simulink model "MASc_AndriyPredmyrskyy_SAC"  (R2020a)
settings: Solver=FixedStepAuto  StartTime=0.0  StopTime=tsim  FixedStep=baseRate  RelTol=1e-3  EnableMultiTasking=on
values from neighbouring files (symbols this model uses):
  Amp1off = 0.2    [Run_Initializer.m]
  Amp2off = 0.1    [Run_Initializer.m]
  baseRate = 0.05    [Run_Initializer.m]
  BLACKMass = 12.3341    [LoadResults.m]    (also in Run_Initializer.m = model_param(3))
  Cmout = [eye(3,3),zeros(3,3)]    [Run_Initializer.m]    (also in SimpleSAC.m = [alpha*eye(3,3),eye(3,3)])
  D = 0    [OptimizationPlots.m]    (also in OptimizeSAC_DE.m; OptimizeSAC_DE_CHANGE.m; OptimizeSAC_PSO.m; SADE_OptimizationForSAC.m)
  drop_states_BLACK = [2.3,1.5,0.176047682762146]    [Run_Initializer.m]
  drop_states_BLUE = [ xLength/2+0.9; yLength/2+0.5; 0]    [Run_Initializer.m]
  drop_states_RED = [2.60644311523438,1.21791186523438,3.08142089843750]    [Run_Initializer.m]
  F_thrusters_BLACK = 0.25.*ones(8,1)    [Run_Initializer.m]
  F_thrusters_BLUE = 0.25.*ones(8,1)    [Run_Initializer.m]
  F_thrusters_RED = 0.25.*ones(8,1)    [Run_Initializer.m]
  GeI = X(2,Best_i).*eye(3)    [OptimizeSAC_DE.m]    (also in OptimizeSAC_DE_CHANGE.m; OptimizeSAC_PSO.m = pos(besti,5).*eye(3); RunAllOptimizations.m = Init.GeI; SADE_OptimizationForSAC.m)
  GeP = X(1,Best_i).*eye(3)    [OptimizeSAC_DE.m]    (also in OptimizeSAC_DE_CHANGE.m; OptimizeSAC_PSO.m = pos(besti,1).*eye(3); RunAllOptimizations.m = Init.GeP; SADE_OptimizationForSAC.m)
  GuI = X(4,Best_i).*eye(3)    [OptimizeSAC_DE.m]    (also in OptimizeSAC_DE_CHANGE.m; OptimizeSAC_PSO.m = pos(besti,8).*eye(3); RunAllOptimizations.m = Init.GuI; SADE_OptimizationForSAC.m)
  GuP = X(3,Best_i).*eye(3)    [OptimizeSAC_DE.m]    (also in OptimizeSAC_DE_CHANGE.m; OptimizeSAC_PSO.m = pos(besti,4).*eye(3); RunAllOptimizations.m = Init.GuP; SADE_OptimizationForSAC.m)
  GxI = blkdiag(X(7,Best_i).*eye(3),X(8,Best_i).*eye(3))    [OptimizeSAC_DE.m]    (also in OptimizeSAC_DE_CHANGE.m = X(6,Best_i).*eye(6); OptimizeSAC_PSO.m = blkdiag(pos(besti,6).*eye(3),pos(besti,7).*eye(3)); RunAllOptimizations.m = Init.GxI; SADE_OptimizationForSAC.m)
  GxP = blkdiag(X(5,Best_i).*eye(3),X(6,Best_i).*eye(3))    [OptimizeSAC_DE.m]    (also in OptimizeSAC_DE_CHANGE.m = X(5,Best_i).*eye(6); OptimizeSAC_PSO.m = blkdiag(pos(besti,2).*eye(3),pos(besti,3).*eye(3)); RunAllOptimizations.m = Init.GxP; SADE_OptimizationForSAC.m)
  GzI = 1e0.*eye(12)    [Run_Initializer.m]
  GzP = 0e-2.*eye(12)    [Run_Initializer.m]
  home_states_BLACK = LastPosition    [Run_Initializer.m]
  home_states_BLUE = [ xLength/2-0.9; yLength/2+0.5; 0]    [Run_Initializer.m]
  home_states_RED = [ xLength/2+0.7; yLength/2; 0]    [Run_Initializer.m]
  init_states_BLACK = FirstPosition    [Run_Initializer.m]
  init_states_BLUE = [ xLength/2+0.9; yLength/2+0.5; 0]    [Run_Initializer.m]
  init_states_RED = [ xLength/2+0.7; yLength/2; 0]    [Run_Initializer.m]
  K = 3    [Run_Initializer.m]    (also in cycloid.m)
  K_Force = 1    [Run_Initializer.m]
  Kd_Force = 3    [Run_Initializer.m]
  Kd_tb = 0.4    [Run_Initializer.m]
  Kd_tblue = 0.4    [Run_Initializer.m]
  Kd_tr = 0.4    [Run_Initializer.m]
  Kd_xb = 5    [Run_Initializer.m]
  Kd_xblue = 5    [Run_Initializer.m]
  Kd_xr = 5    [Run_Initializer.m]
  Kd_yb = 5    [Run_Initializer.m]
  Kd_yblue = 5    [Run_Initializer.m]
  Kd_yr = 5    [Run_Initializer.m]
  KeI0 = 0.*[   0.1063   -0.0058         0 ... (first row only)    [Run_Initializer.m]    (also in SimpleSAC.m = zeros(3))
  Kp_tb = 0.1    [Run_Initializer.m]
  Kp_tblue = 0.1    [Run_Initializer.m]
  Kp_tr = 0.1    [Run_Initializer.m]
  Kp_xb = 2    [Run_Initializer.m]
  Kp_xblue = 2    [Run_Initializer.m]
  Kp_xr = 2    [Run_Initializer.m]
  Kp_yb = 2    [Run_Initializer.m]
  Kp_yblue = 2    [Run_Initializer.m]
  Kp_yr = 2    [Run_Initializer.m]
  KuI0 = 0.*0.2193*[1,0,0;0,1,0;0,0,0]    [Run_Initializer.m]    (also in SimpleSAC.m = zeros(3))
  KxI0 = 0.*[-0.2193*eye(3),-3.2891*eye(3)]    [Run_Initializer.m]    (also in SimpleSAC.m = zeros(3,6))
  KzI0 = zeros(3,12)    [Run_Initializer.m]
  noise_variance_BLACK = 0    [Run_Initializer.m]
  noise_variance_BLUE = 0    [Run_Initializer.m]
  noise_variance_RED = 0    [Run_Initializer.m]
  omega = 0.03    [LoadResults.m]    (also in OptimizeSAC_PSO.m = 0.2; Run_Initializer.m = 0.06; SPSO_OptimizationForSAC.m = 0.2; SimpleSAC.m = sqrt(Force./(Mass*Radius)))
  omega1off = 0.03    [Run_Initializer.m]
  omega2off = 0.06    [Run_Initializer.m]
  Phase0_End = Phase0_Duration    (= 10)    [Run_Initializer.m]
  Phase1_End = Phase0_Duration + Phase1_Duration    (= 15)    [Run_Initializer.m]
  phase1off = 2*pi + 3-2+1.0654    (= 8.34858530718)    [Run_Initializer.m]
  Phase2_End = Phase0_Duration + Phase1_Duration +                                   Phase2_Duration    (= 35)    [Run_Initializer.m]
  phase2off = mod(pi^66,2*pi)    [Run_Initializer.m]
  Phase3_End = Phase0_Duration + Phase1_Duration +                                   Phase2_Duration + Phase3_Duration    (= 246)    [Run_Initializer.m]
  Phase3_SubPhase1_End = Phase2_End + Phase3_SubPhase1_Duration    (= 40)    [Run_Initializer.m]
  Phase3_SubPhase2_End = Phase2_End + Phase3_SubPhase1_Duration +                                   Phase3_SubPhase2_Duration    (= 45)    [Run_Initializer.m]
  Phase3_SubPhase3_End = Phase2_End + Phase3_SubPhase1_Duration +                                   Phase3_SubPhase2_Duration +                                  Phase3_SubPhase3_Duration    (= 46)    [Run_Initializer.m]
  Phase3_SubPhase4_End = Phase2_End + Phase3_SubPhase1_Duration +                                   Phase3_SubPhase2_Duration +                                  Phase3_SubPhase3_Duration +                                  Phase3_SubPhase4_Duration    [Run_Initializer.m]
  Phase4_End = Phase0_Duration + Phase1_Duration +                                   Phase2_Duration + Phase3_Duration +                                   Phase4_Duration    (= 266)    [Run_Initializer.m]
  Phase5_End = Phase0_Duration + Phase1_Duration +                                   Phase2_Duration + Phase3_Duration +                                   Phase4_Duration + Phase5_Duration    (= 271)    [Run_Initializer.m]
  platformSelection = 1    [OptimizationPlots.m]    (also in OptimizeSAC_DE.m; OptimizeSAC_DE_CHANGE.m; OptimizeSAC_PSO.m; SADE_OptimizationForSAC.m)
  serverRate = 0.1    [Run_Initializer.m]    (also in SimpleSAC.m)
  sigma_eI = X(9,Best_i)    [OptimizeSAC_DE.m]    (also in OptimizeSAC_DE_CHANGE.m = X(7,Best_i); OptimizeSAC_PSO.m = pos(besti,9); RunAllOptimizations.m = Init.sigma_eI; SADE_OptimizationForSAC.m)
  sigma_uI = X(10,Best_i)    [OptimizeSAC_DE.m]    (also in OptimizeSAC_DE_CHANGE.m = X(8,Best_i); OptimizeSAC_PSO.m = pos(besti,11); RunAllOptimizations.m = Init.sigma_uI; SADE_OptimizationForSAC.m)
  sigma_xI = X(11,Best_i)    [OptimizeSAC_DE.m]    (also in OptimizeSAC_DE_CHANGE.m = X(9,Best_i); OptimizeSAC_PSO.m = pos(besti,10); RunAllOptimizations.m = Init.sigma_xI; SADE_OptimizationForSAC.m)
  sigma_zI = 0    [Run_Initializer.m]
  sysd1 = c2d(sys,baseRate,opt)    [Run_Initializer.m]    (also in SimpleSAC.m = c2d(sys,serverRate,opt))
  sysd2 = c2d(sysInverse,baseRate,opt)    [Run_Initializer.m]
  thruster_dist2CG_BLACK = [83.42;-52.58;55.94;-60.05;54.08;-53.92;77.06;-55.94]    [Run_Initializer.m]
  thruster_dist2CG_BLUE = [83.42;-52.58;55.94;-60.05;54.08;-53.92;77.06;-55.94]    [Run_Initializer.m]
  thruster_dist2CG_RED = [49.92;-78.08;70.46;-63.54;81.08;-50.42;57.44;-75.96]    [Run_Initializer.m]
  xm2_ini = -(sysd2.D(1,1).*xm_ini(1:3))./(sysd2.C(1,1))    [Run_Initializer.m]
  xm_ini = [FirstPosition(1), FirstPosition(2), 0, 0, 0, 0]'    [Run_Initializer.m]    (also in SimpleSAC.m = [0, 0, 0, 0, 0, 0]')
undefined symbols (not defined in the file or in its folder): DiscIntNeverNeededParam, G3, simMode, WhoAmI
libraries: dspstat3 x18, simulink x12, raspberrypiBasiclib x10, dspsigops x9, embdlinuxlib x8, mspfiltlib x3, dsparch4 x3, peGeneralControl x3, eeGeneralControl x3, dspswit3 x2, MainLibrary x2, sensehatlib x1
(part 11 of 11)

== matlab function MASc_AndriyPredmyrskyy_SAC/From Torque, Command RW/Change RED Behavior/Calculate Saturated RPM Signal/Calculate RW RPM Increment ==
  data: Tz_Sat input; dRPM_RW output
function dRPM_RW = Calc_RW_RPM(Tz_Sat)

dRPM_RW =  (Tz_Sat/0.007244720)*(60/2/pi)*0.1;

end

== matlab function MASc_AndriyPredmyrskyy_SAC/From Torque, Command RW/Change RED Behavior/Wheel RPM to PWM/Check if RW is Ready ==
  data: Status input; EnableSig output; WheelRPM_In input; WheelRPM_Out output
function [EnableSig, WheelRPM_Out] = Check_Wheel_Status(Status, WheelRPM_In)

if Status == 0
    EnableSig    = 1;
    WheelRPM_Out = WheelRPM_In;
else
    EnableSig    = 0;
    WheelRPM_Out = 0;
end

end

== matlab function MASc_AndriyPredmyrskyy_SAC/From Torque, Command RW/Change RED Behavior/Wheel RPM to PWM/Get RW Direction ==
  data: MotorRPM_Sat input; WheelDirection output
function WheelDirection = GetDirection(MotorRPM_Sat)

if MotorRPM_Sat > 0
    WheelDirection = 0;
else
    WheelDirection = 1;
end
        
end

== matlab function MASc_AndriyPredmyrskyy_SAC/From Torque, Command RW/Change RED Behavior/Wheel RPM to PWM/RPM to PWM Value ==
  data: MotorRPM_Sat input; MotorPWM output
function MotorPWM = RPM2PWM(MotorRPM_Sat)

PWMRange = 0.9-0.1;

MotorPWM = ((MotorRPM_Sat*PWMRange)/7000) + 0.1;

end

== matlab function MASc_AndriyPredmyrskyy_SAC/Phase #3: Experiment/Change RED Behavior/Sub-Phase #4/MATLAB Function ==
  data: t input; x output; xLength parameter
function x = fcn(t, xLength)

x = 0.7*cos((0.104719755/2)*t) + xLength/2;

end

== matlab function MASc_AndriyPredmyrskyy_SAC/From Force//Torque to PWM Signal/Change BLUE Behavior/Calculate Thruster ON//OFF/MATLAB Function ==
  data: H output; thruster_dist2CG_BLUE parameter; F_thrusters_BLUE parameter
function H = MakeH(thruster_dist2CG_BLUE,F_thrusters_BLUE)

Vec1 = [ -1
         -1
          0 
          0
          1
          1
          0
          0 ];
      
Vec2 = [  0
          0
          1
          1
          0
          0
         -1
         -1 ];
     
Vec3 = thruster_dist2CG_BLUE./1000;

Mat1 = [Vec1, Vec2, Vec3]';

Mat2 = diag((F_thrusters_BLUE./2));

H    = Mat1*Mat2;

end

== matlab function MASc_AndriyPredmyrskyy_SAC/Phase #3: Experiment/Change RED Behavior/Sub-Phase #4/MATLAB Function1 ==
  data: t input; y output; yLength parameter
function y = fcn(t, yLength)

y = 0.7*sin((0.104719755/2)*t) + yLength/2;

end

== matlab function MASc_AndriyPredmyrskyy_SAC/Phase #3: Experiment/Change BLACK Behavior/Sub-Phase #4/Hough Control/MATLAB Function4 ==
  data: Oy input; e_out output; e_in input
function e_out = fcn(Oy, e_in)

a = sign(Oy'*e_in);
e_out = -a*norm(e_in);

== matlab function MASc_AndriyPredmyrskyy_SAC/Gyroscope & Acceleration Algorithms/Change RED Behavior/Create Rotation Matrix ==
  data: Rz input; C_Ib output
function C_Ib = RotateFrame(Rz)

C_bI = [  cos(Rz) sin(Rz)
         -sin(Rz) cos(Rz) ];

C_Ib = inv(C_bI);

end

== matlab function MASc_AndriyPredmyrskyy_SAC/Gyroscope & Acceleration Algorithms/Change BLACK Behavior/Create Rotation Matrix ==
  data: Rz input; C_Ib output
function C_Ib = RotateFrame(Rz)

C_bI = [  cos(Rz) sin(Rz)
         -sin(Rz) cos(Rz) ];

C_Ib = inv(C_bI);

end

== matlab function MASc_AndriyPredmyrskyy_SAC/Gyroscope & Acceleration Algorithms/Change RED Behavior/ChangeOrientation ==
  data: u input; y output
function y = ChangeOrientation(u)

y = rotz(-90)*u';

== matlab function MASc_AndriyPredmyrskyy_SAC/Gyroscope & Acceleration Algorithms/Change BLACK Behavior/ChangeOrientation ==
  data: u input; y output
function y = ChangeOrientation(u)

y = rotz(-90)*u';

== matlab function MASc_AndriyPredmyrskyy_SAC/Gyroscope & Acceleration Algorithms/Change BLUE Behavior/ChangeOrientation ==
  data: u input; y output
function y = ChangeOrientation(u)

y = rotz(-90)*u';

== matlab function MASc_AndriyPredmyrskyy_SAC/Gyroscope & Acceleration Algorithms/Change BLUE Behavior/Create Rotation Matrix ==
  data: Rz input; C_Ib output
function C_Ib = RotateFrame(Rz)

C_bI = [  cos(Rz) sin(Rz)
         -sin(Rz) cos(Rz) ];

C_Ib = inv(C_bI);

end

== matlab function MASc_AndriyPredmyrskyy_SAC/From Force//Torque to PWM Signal/Change BLUE Behavior/Calculate Thruster ON//OFF/MATLAB Function1 ==
  data: H output; thruster_dist2CG_BLUE parameter; F_thrusters_BLUE parameter
function H = MakeH(thruster_dist2CG_BLUE,F_thrusters_BLUE)

Vec1 = [ -1
         -1
          0 
          0
          1
          1
          0
          0 ];
      
Vec2 = [  0
          0
          1
          1
          0
          0
         -1
         -1 ];
     
Vec3 = thruster_dist2CG_BLUE./1000;

Mat1 = [Vec1, Vec2, Vec3]';

Mat2 = diag((F_thrusters_BLUE./2));

H    = Mat1*Mat2;

end

== matlab function MASc_AndriyPredmyrskyy_SAC/From Force//Torque to PWM Signal/Change BLUE Behavior/Calculate Thruster ON//OFF/MATLAB Function2 ==
  data: ThrustPer_Final output; ThrustPer input
function ThrustPer_Final  = ThrusterSat(ThrustPer)

ValveTime       = 0.007;
TControl        = 0.1;
ThrustPer_Final = zeros(8,1);

if max(ThrustPer) > 1
    ThrustPer_Sat = ThrustPer/max(ThrustPer);
else
    ThrustPer_Sat = ThrustPer;
end

for i = 1:8
    if ThrustPer_Sat(i) > ValveTime/TControl 
        ThrustPer_Final(i) = ThrustPer_Sat(i);
    else
        ThrustPer_Final(i) = 0;
    end
end
   

end

== matlab function MASc_AndriyPredmyrskyy_SAC/From Force//Torque to PWM Signal/Change BLUE Behavior/Calculate Thruster ON//OFF/Rotate Forces to Inertial/Create Rotation Matrix ==
  data: Rz input; C_Ib output
function C_Ib = RotateFrame(Rz)

C_bI = [  cos(Rz) sin(Rz)
         -sin(Rz) cos(Rz) ];

C_Ib = inv(C_bI);

end

== matlab function MASc_AndriyPredmyrskyy_SAC/From Force//Torque to PWM Signal/Change BLUE Behavior/Rotate Forces to Body/Create Rotation Matrix ==
  data: Rz input; C_bI output
function C_bI = RotateFrame(Rz)

C_bI = [  cos(Rz) sin(Rz)
         -sin(Rz) cos(Rz) ];

end

== matlab function MASc_AndriyPredmyrskyy_SAC/Phase #2: Move to Initial Position/Change BLACK Behavior/Hough Control/MATLAB Function2 ==
  data: Oy output; z input; Ox output
function [Oy, Ox]   = C3( z )
%C3 gives the rotation matrix about the z-axis for an angle 'z'
%   z - the angle about the z-axis which you rotate
%   A - the rotation matrix

Ox = [cos(z) sin(z); -sin(z) cos(z)]*[1;0];
Oy = [cos(z) sin(z); -sin(z) cos(z)]*[0;1];
end
